simulink model "P7Simulink"  (R2025b)
settings: Solver=VariableStepAuto  StartTime=0.0  StopTime=10.0  RelTol=1e-3
settings Model: Creator=juani  LastModifiedBy=juani

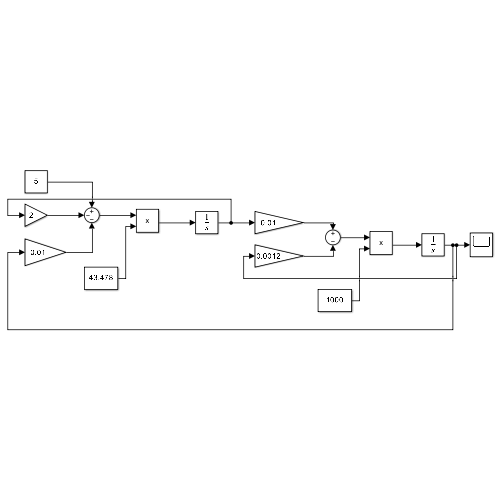
[thumbnail: Simulink's stored preview of the top-level diagram]
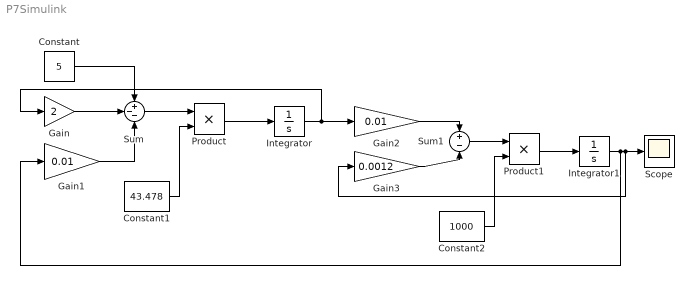
== system P7Simulink ==
  Constant : Constant  Value=5
  Constant1 : Constant  Value=43.478
  Constant2 : Constant  Value=1000
  Gain : Gain  Gain=2
  Gain1 : Gain  Gain=0.01
  Gain2 : Gain  Gain=0.01
  Gain3 : Gain  Gain=0.0012
  Integrator : Integrator
  Integrator1 : Integrator
  Product : Product
  Product1 : Product
  Scope : Scope
      settings: ActiveDisplayYMinimum=-2.5000247375850186  ActiveDisplayYMaximum=22.500222638265171
  Sum : Sum  Inputs=+--
  Sum1 : Sum  Inputs=+-
  wires:
  Constant/1 -> Sum/1
  Gain/1 -> Sum/2
  Gain1/1 -> Sum/3
  Sum/1 -> Product/1
  Constant1/1 -> Product/2
  Product/1 -> Integrator/1
  Integrator/1 -> Gain/1, Gain2/1
  Gain2/1 -> Sum1/1
  Gain3/1 -> Sum1/2
  Constant2/1 -> Product1/2
  Sum1/1 -> Product1/1
  Product1/1 -> Integrator1/1
  Integrator1/1 -> Gain1/1, Gain3/1, Scope/1
